simulink model "non_linear_PID_tune"  (R2020b)
settings: Solver=FixedStepAuto  StartTime=0.0  StopTime=3  FixedStep=0.0001  RelTol=1e-3
model workspace (MAT data in the model file):
  Kd = 0.7104640041
  Ki = 2.17380443913
  Kp = 96.3943895939
libraries: checkpacklib x1
settings Model: OrderedModelArguments=off  Creator=morro  LastModifiedBy=morro
settings DataIOCC: ReturnWorkspaceOutputsName=SDOSimTest_Log

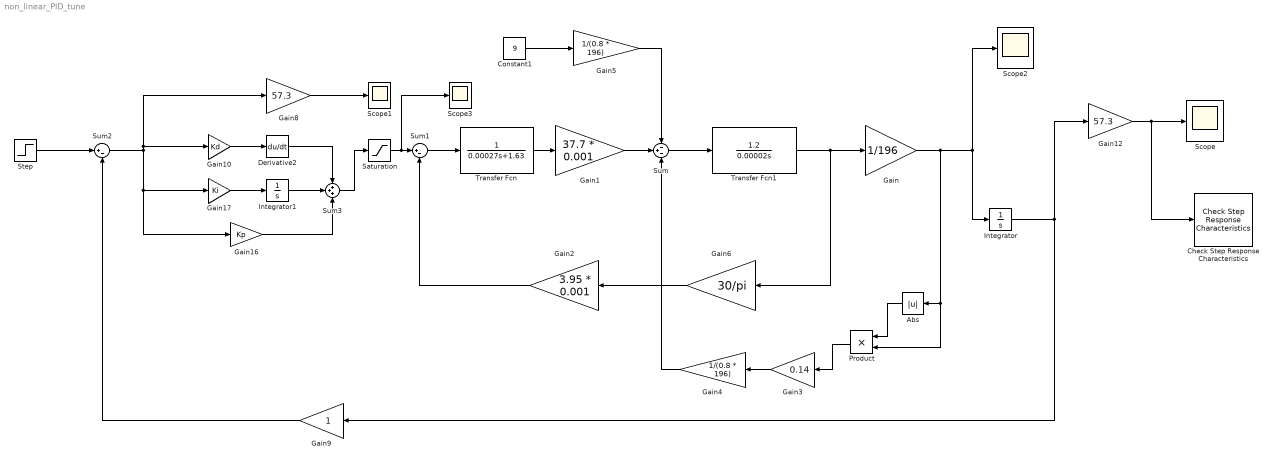
== system non_linear_PID_tune ==
  Abs : Abs
  Check Step Response Characteristics : checkpacklib/Check Step Response  Characteristics  InstantiateOnLoad=on  enabled=off  stopWhenAssertionFail=off  export=off  ViewDlgPos=[]  OpenViewOnLoad=off  LaunchViewOnOpen=off  TimeUnits=seconds  EnableStepResponseBound=on  InitialValue=0  FinalValue=100  StepTime=1  RiseTime=0.6  PercentRise=80  SettlingTime=0.8  PercentSettling=0.9  PercentOvershoot=0.9  PercentUndershoot=2
      settings: SourceProductBaseCode=CT,ID,MT,SO
  Constant1 : Constant  Value=9
  Derivative2 : Derivative
  Gain : Gain  Gain=1/196
  Gain1 : Gain  Gain=37.7 * 0.001
  Gain10 : Gain  Gain=Kd
  Gain12 : Gain  Gain=57.3
  Gain16 : Gain  Gain=Kp
  Gain17 : Gain  Gain=Ki
  Gain2 : Gain  Gain=3.95 * 0.001
  Gain3 : Gain  Gain=0.14
  Gain4 : Gain  Gain=1/(0.8 * 196)
  Gain5 : Gain  Gain=1/(0.8 * 196)
  Gain6 : Gain  Gain=30/pi
  Gain8 : Gain  Gain=57.3
  Gain9 : Gain
  Integrator : Integrator  InitialCondition=1e-7
  Integrator1 : Integrator  InitialCondition=1e-7
  Product : Product
  Saturation : Saturate  UpperLimit=27  LowerLimit=-27
  Scope{,1..3} (4 alike) : Scope
  Step : Step  After=100/57.3  SampleTime=0
  Sum : Sum  Inputs=-+-
  Sum1 : Sum  Inputs=|+-
  Sum2 : Sum  Inputs=|+-
  Sum3 : Sum  Inputs=+++
  Transfer Fcn : TransferFcn  Denominator=[0.00027 1.63]
  Transfer Fcn1 : TransferFcn  Numerator=[1.2]  Denominator=[0.00002 0]
  wires:
  Gain1/1 -> Sum/2
  Constant1/1 -> Gain5/1
  Gain4/1 -> Sum/3
  Product/1 -> Gain3/1
  Abs/1 -> Product/1
  Step/1 -> Sum2/1
  Gain6/1 -> Gain2/1
  Transfer Fcn/1 -> Gain1/1
  Gain2/1 -> Sum1/2
  Transfer Fcn1/1 -> Gain6/1, Gain/1
  Gain5/1 -> Sum/1
  Gain8/1 -> Scope1/1
  Gain12/1 -> Check Step Response Characteristics/1, Scope/1
  Integrator/1 -> Gain9/1, Gain12/1
  Sum/1 -> Transfer Fcn1/1
  Gain9/1 -> Sum2/2
  Gain3/1 -> Gain4/1
  Sum2/1 -> Gain10/1, Gain8/1, Gain16/1, Gain17/1
  Gain/1 -> Product/2, Abs/1, Integrator/1, Scope2/1
  Gain10/1 -> Derivative2/1
  Gain17/1 -> Integrator1/1
  Gain16/1 -> Sum3/3
  Integrator1/1 -> Sum3/2
  Derivative2/1 -> Sum3/1
  Sum1/1 -> Transfer Fcn/1
  Saturation/1 -> Scope3/1, Sum1/1
  Sum3/1 -> Saturation/1
